simulink model "Ec_Diferencias"  (R2023b)
settings: Solver=VariableStepAuto  StartTime=0.0  StopTime=10.0  RelTol=1e-3
settings Model: Creator=carlo  LastModifiedBy=carlo

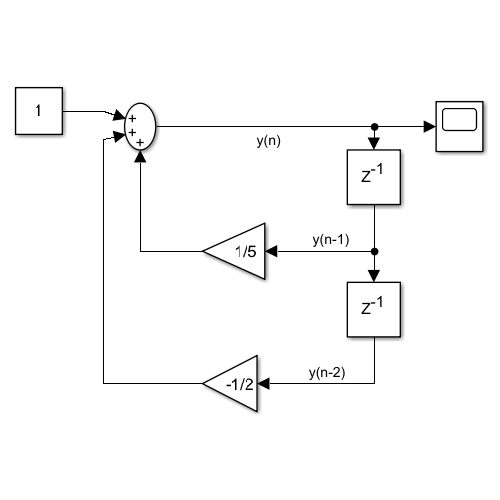
[thumbnail: Simulink's stored preview of the top-level diagram]
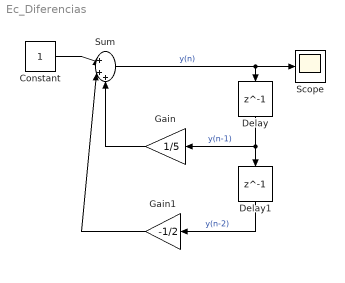
== system Ec_Diferencias ==
  Constant : Constant  SampleTime=1
  Delay : Delay  DelayLength=1
  Delay1 : Delay  DelayLength=1
  Gain : Gain  Gain=1/5
  Gain1 : Gain  Gain=-1/2
  Scope : Scope
  Sum : Sum  Inputs=|+++
  wires:
  Delay/1 -> Gain/1, Delay1/1  "y(n-1)"
  Sum/1 -> Scope/1, Delay/1  "y(n)"
  Delay1/1 -> Gain1/1  "y(n-2)"
  Gain/1 -> Sum/3
  Gain1/1 -> Sum/2
  Constant/1 -> Sum/1
